simulink model "kinematics"  (Simulink 7.9)
settings: Solver=ode3  StartTime=0.0  StopTime=10.0  FixedStep=0.005  RelTol=1e-5
values from neighbouring files (symbols this model uses):
  initial_ee_eta = zeros(1,6)    [kinematic_parameters.m]
  initial_eta = [0,0,0,0,0,0]    [kinematic_parameters.m]
  initial_eta1 = initial_eta(1:3)    [kinematic_parameters.m]
  initial_eta2 = initial_eta(4:6)    [kinematic_parameters.m]
  initial_q = [0,20*d2r,-(20+25)*d2r,25*d2r,-90*d2r,0]    [kinematic_parameters.m]
  v_ee_c = [0.1,0,0,0,0.2,0]    [kinematic_parameters.m]
undefined symbols (not defined in the file or in its folder): a, alpha, d, qmax, qmin
libraries: simulink x3
settings Model: Creator=simena  LastModifiedBy=simena
settings OptimizationCC: EfficientMapNaN2IntZero=off
settings HardwareCC: TargetIntDivRoundTo=Zero  TargetEndianess=LittleEndian  TargetHWDeviceType=MATLAB Host  ProdEqTarget=off
settings CodeAppCC: MaxIdLength=128
settings GRTTargetCC: CombineOutputUpdateFcns=off  GRTInterface=on

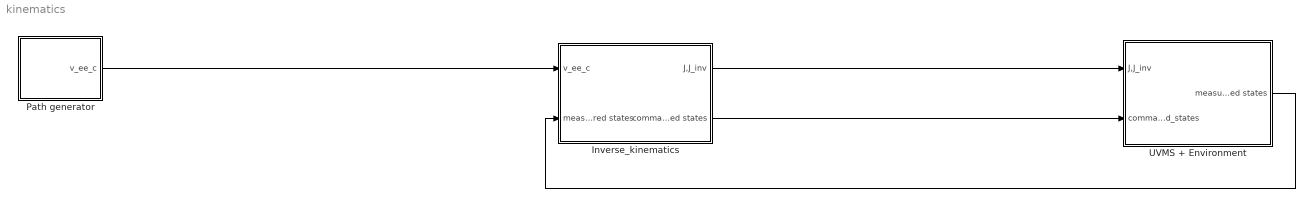
== system kinematics ==
  "Inverse_kinematics " : Subsystem
  Path generator : Subsystem
  UVMS + Environment : Subsystem
  wires:
  Path generator/1(v_ee_c) -> "Inverse_kinematics "/1(v_ee_c)
  "Inverse_kinematics "/1(J,J_inv) -> UVMS + Environment/1(J,J_inv)
  "Inverse_kinematics "/2(commanded states) -> UVMS + Environment/2(commanded_states)
  UVMS + Environment/1(measured states) -> "Inverse_kinematics "/2(measured states)

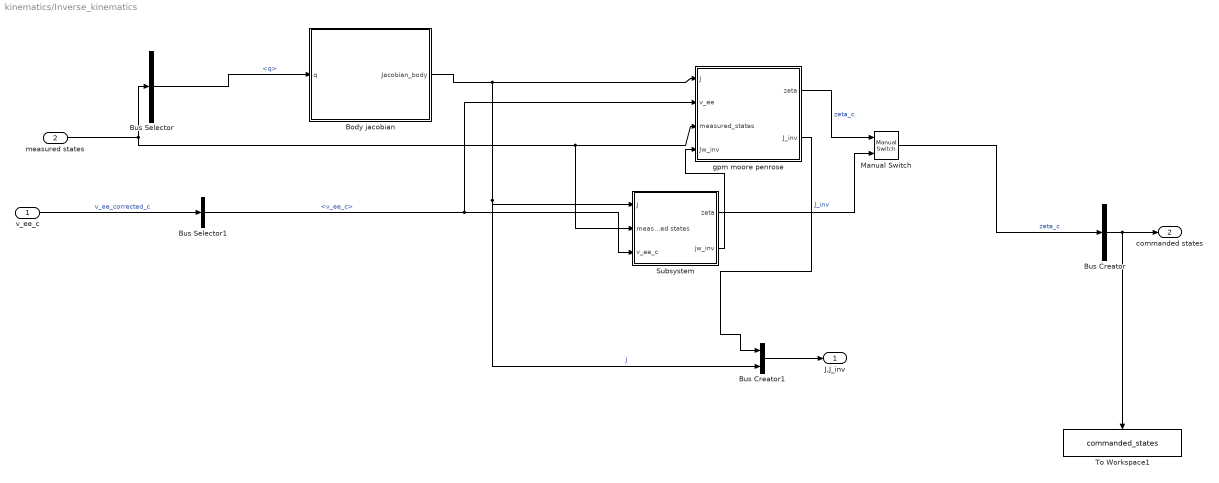
== system kinematics/Inverse_kinematics  ==
  v_ee_c : Inport
  measured states : Inport  Port=2
  Body jacobian : MATLAB Function  TreatAsAtomicUnit=on
  Bus Creator : BusCreator  Inputs=1
  Bus Creator1 : BusCreator  Inputs=2
  Bus Selector : BusSelector  OutputSignals=xi.q
  Bus Selector1 : BusSelector  OutputSignals=v_ee_c
  Manual Switch : simulink/Signal Routing/Manual Switch  sw=0  action=0  varsize=off
  Subsystem : Subsystem
  To Workspace1 : ToWorkspace  VariableName=commanded_states  SampleTime=-1  SaveFormat=Timeseries
  gpm moore penrose : Subsystem
  J,J_inv : Outport
  commanded states : Outport  Port=2
  wires:
  measured states/1 -> Bus Selector/1, gpm moore penrose/3(measured_states), Subsystem/2(measured states)
  Bus Creator/1 -> commanded states/1, To Workspace1/1
  Bus Creator1/1 -> J,J_inv/1
  gpm moore penrose/2(J_inv) -> Bus Creator1/1  "J_inv"
  v_ee_c/1 -> Bus Selector1/1  "v_ee_corrected_c"
  Body jacobian/1(Jacobian_body) -> gpm moore penrose/1(J), Bus Creator1/2, Subsystem/1(J)  "J"
  Bus Selector/1 -> Body jacobian/1(q)  "<q>"
  gpm moore penrose/1(zeta) -> Manual Switch/1  "zeta_c"
  Manual Switch/1 -> Bus Creator/1  "zeta_c"
  Subsystem/1(zeta) -> Manual Switch/2
  Bus Selector1/1 -> Subsystem/3(v_ee_c), gpm moore penrose/2(v_ee)  "<v_ee_c>"
  Subsystem/2(jw_inv) -> gpm moore penrose/4(Jw_inv)

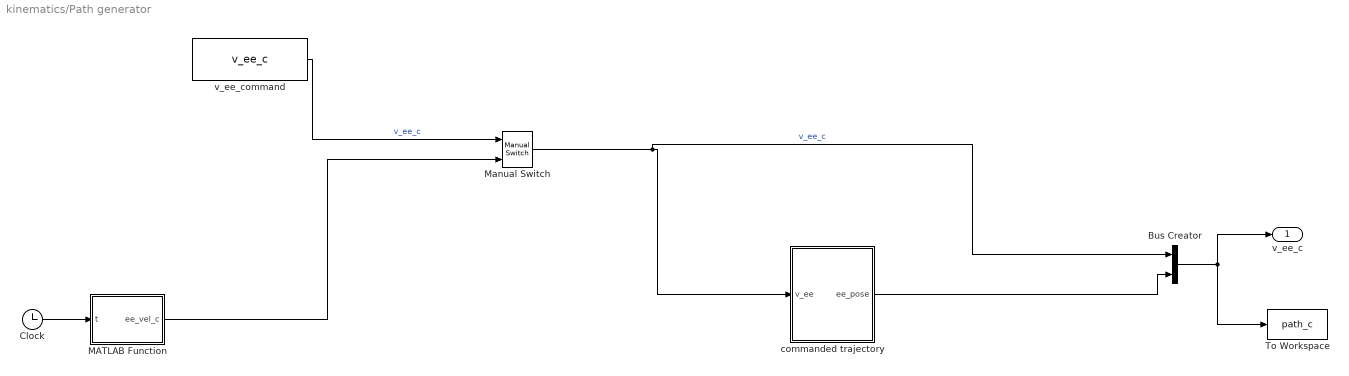
== system kinematics/Path generator ==
  Bus Creator : BusCreator  Inputs=2
  Clock : Clock
  MATLAB Function : MATLAB Function  TreatAsAtomicUnit=on
  Manual Switch : simulink/Signal Routing/Manual Switch  sw=0  action=0  varsize=off
  To Workspace : ToWorkspace  VariableName=path_c  SampleTime=-1  SaveFormat=Timeseries
  commanded trajectory : Subsystem
  v_ee_command : Constant  Value=v_ee_c
  v_ee_c : Outport
  wires:
  commanded trajectory/1(ee_pose) -> Bus Creator/2
  Bus Creator/1 -> v_ee_c/1, To Workspace/1
  v_ee_command/1 -> Manual Switch/1  "v_ee_c"
  Manual Switch/1 -> commanded trajectory/1(v_ee), Bus Creator/1  "v_ee_c"
  Clock/1 -> MATLAB Function/1(t)
  MATLAB Function/1(ee_vel_c) -> Manual Switch/2

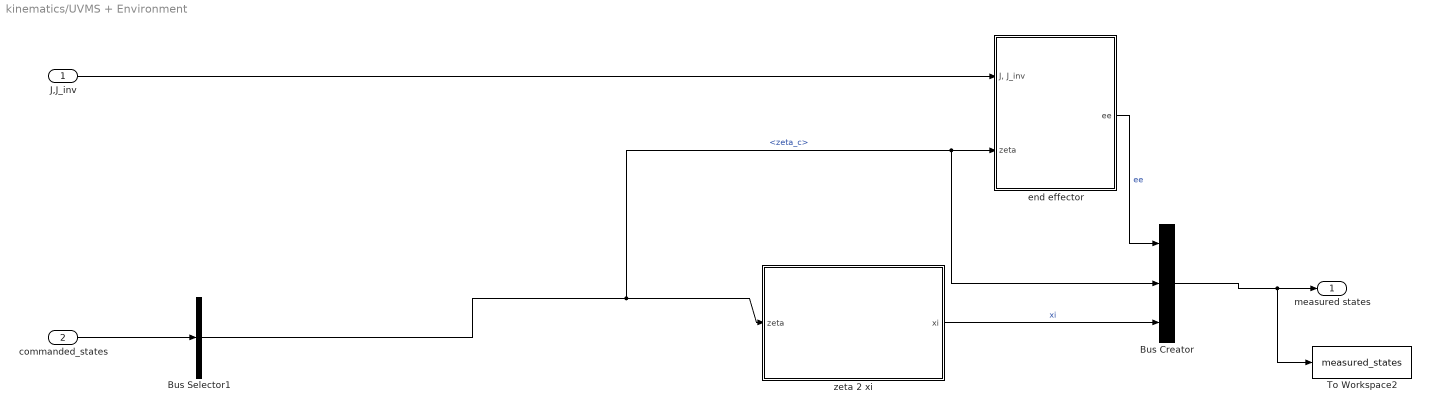
== system kinematics/UVMS + Environment ==
  J,J_inv : Inport
  commanded_states : Inport  Port=2
  Bus Creator : BusCreator  Inputs=3
  Bus Selector1 : BusSelector  OutputSignals=zeta_c
  To Workspace2 : ToWorkspace  VariableName=measured_states  SampleTime=-1  SaveFormat=Timeseries
  end effector : Subsystem
  zeta 2 xi : Subsystem
  measured states : Outport
  wires:
  zeta 2 xi/1(xi) -> Bus Creator/3  "xi"
  J,J_inv/1 -> end effector/1("J, J_inv")
  end effector/1(ee) -> Bus Creator/1  "ee"
  commanded_states/1 -> Bus Selector1/1
  Bus Creator/1 -> measured states/1, To Workspace2/1
  Bus Selector1/1 -> zeta 2 xi/1(zeta), end effector/2(zeta), Bus Creator/2  "<zeta_c>"

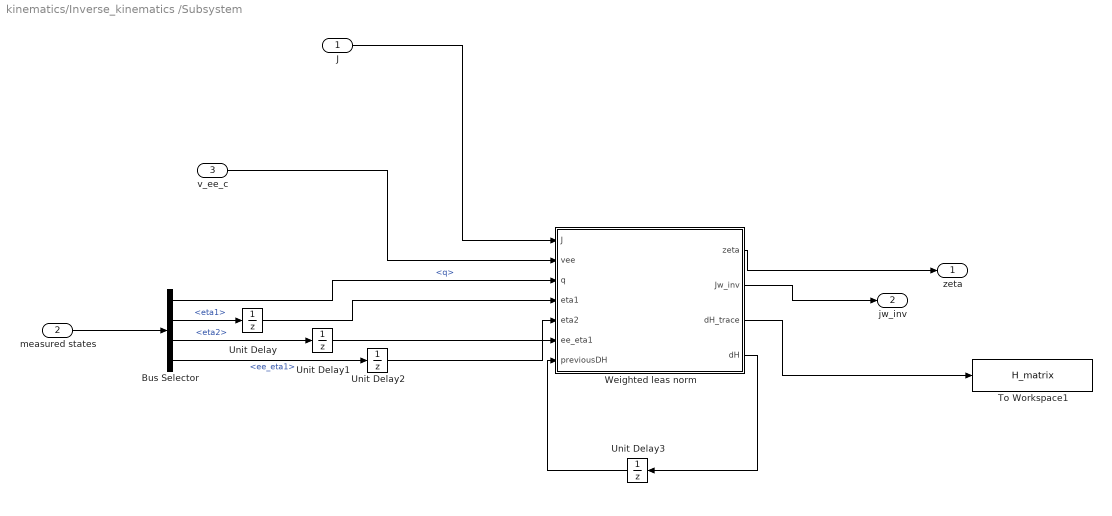
== system kinematics/Inverse_kinematics /Subsystem ==
  J : Inport
  measured states : Inport  Port=2
  v_ee_c : Inport  Port=3
  Bus Selector : BusSelector  OutputSignals=xi.q,xi.eta1,xi.eta2,ee.ee_eta1
  To Workspace1 : ToWorkspace  VariableName=H_matrix  SampleTime=-1  SaveFormat=Timeseries
  Unit Delay : UnitDelay  X0=initial_eta1  SampleTime=-1
  Unit Delay1 : UnitDelay  X0=initial_eta2  SampleTime=-1
  Unit Delay2 : UnitDelay  X0=initial_ee_eta(4:6)  SampleTime=-1
  Unit Delay3 : UnitDelay  X0=zeros(12,12)  SampleTime=-1
  Weighted leas norm : MATLAB Function  TreatAsAtomicUnit=on
  zeta : Outport
  jw_inv : Outport  Port=2
  wires:
  Weighted leas norm/1(zeta) -> zeta/1
  J/1 -> Weighted leas norm/1(J)
  measured states/1 -> Bus Selector/1
  v_ee_c/1 -> Weighted leas norm/2(vee)
  Bus Selector/1 -> Weighted leas norm/3(q)  "<q>"
  Bus Selector/2 -> Unit Delay/1  "<eta1>"
  Bus Selector/3 -> Unit Delay1/1  "<eta2>"
  Bus Selector/4 -> Unit Delay2/1  "<ee_eta1>"
  Unit Delay/1 -> Weighted leas norm/4(eta1)
  Unit Delay1/1 -> Weighted leas norm/5(eta2)
  Unit Delay2/1 -> Weighted leas norm/6(ee_eta1)
  Weighted leas norm/2(Jw_inv) -> jw_inv/1
  Weighted leas norm/3(dH_trace) -> To Workspace1/1
  Weighted leas norm/4(dH) -> Unit Delay3/1
  Unit Delay3/1 -> Weighted leas norm/7(previousDH)

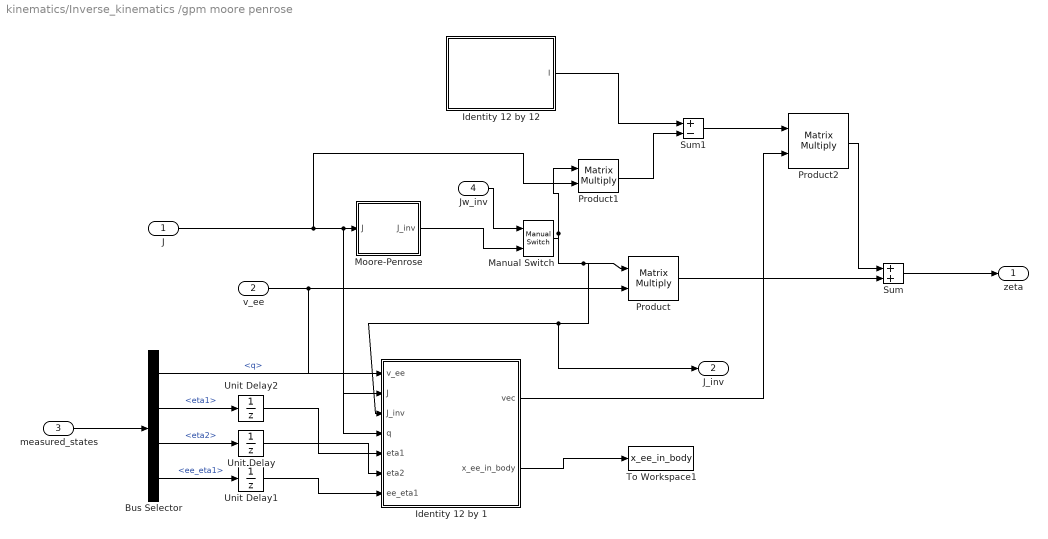
== system kinematics/Inverse_kinematics /gpm moore penrose ==
  J : Inport
  v_ee : Inport  Port=2
  measured_states : Inport  Port=3
  Jw_inv : Inport  Port=4
  Bus Selector : BusSelector  OutputSignals=xi.q,xi.eta1,xi.eta2,ee.ee_eta1
  Identity 12 by 1 : MATLAB Function  TreatAsAtomicUnit=on
  Identity 12 by 12 : MATLAB Function  TreatAsAtomicUnit=on
  Manual Switch : simulink/Signal Routing/Manual Switch  sw=1  action=0  varsize=off
  Moore-Penrose : MATLAB Function  TreatAsAtomicUnit=on
  Product : Product  Multiplication=Matrix(*)  RndMeth=Zero
  Product1 : Product  Multiplication=Matrix(*)  RndMeth=Zero
  Product2 : Product  Multiplication=Matrix(*)  RndMeth=Zero
  Sum : Sum
  Sum1 : Sum  Inputs=+-
  To Workspace1 : ToWorkspace  VariableName=x_ee_in_body  SampleTime=-1  SaveFormat=Timeseries
  Unit Delay : UnitDelay  X0=initial_eta2  SampleTime=-1
  Unit Delay1 : UnitDelay  X0=initial_ee_eta(1:3)  SampleTime=-1
  Unit Delay2 : UnitDelay  X0=initial_eta1  SampleTime=-1
  zeta : Outport
  J_inv : Outport  Port=2
  wires:
  Product/1 -> Sum/2
  Identity 12 by 12/1(I) -> Sum1/1
  Product1/1 -> Sum1/2
  Sum1/1 -> Product2/1
  Product2/1 -> Sum/1
  v_ee/1 -> Product/2, Identity 12 by 1/1(v_ee)
  Sum/1 -> zeta/1
  Identity 12 by 1/1(vec) -> Product2/2
  measured_states/1 -> Bus Selector/1
  Bus Selector/2 -> Unit Delay2/1  "<eta1>"
  Bus Selector/4 -> Unit Delay1/1  "<ee_eta1>"
  Bus Selector/3 -> Unit Delay/1  "<eta2>"
  Bus Selector/1 -> Identity 12 by 1/4(q)  "<q>"
  Unit Delay2/1 -> Identity 12 by 1/5(eta1)
  Unit Delay/1 -> Identity 12 by 1/6(eta2)
  Unit Delay1/1 -> Identity 12 by 1/7(ee_eta1)
  Jw_inv/1 -> Manual Switch/1
  Moore-Penrose/1(J_inv) -> Manual Switch/2
  Manual Switch/1 -> Product1/1, Product/1, Identity 12 by 1/3(J_inv), J_inv/1
  J/1 -> Moore-Penrose/1(J), Identity 12 by 1/2(J), Product1/2
  Identity 12 by 1/2(x_ee_in_body) -> To Workspace1/1

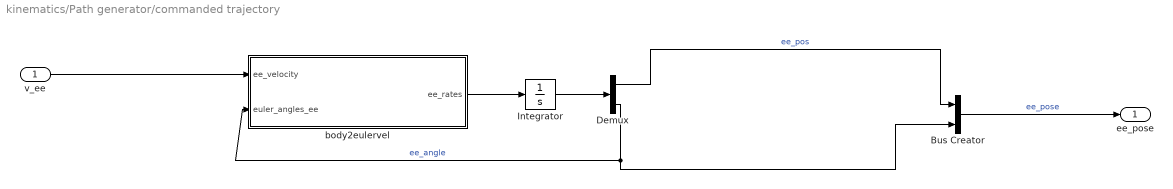
== system kinematics/Path generator/commanded trajectory ==
  v_ee : Inport
  Bus Creator : BusCreator  Inputs=2
  Demux : Demux  Outputs=2
  Integrator : Integrator  InitialCondition=initial_ee_eta
  body2eulervel : MATLAB Function  TreatAsAtomicUnit=on
  ee_pose : Outport
  wires:
  v_ee/1 -> body2eulervel/1(ee_velocity)
  body2eulervel/1(ee_rates) -> Integrator/1
  Integrator/1 -> Demux/1
  Demux/1 -> Bus Creator/1  "ee_pos"
  Demux/2 -> body2eulervel/2(euler_angles_ee), Bus Creator/2  "ee_angle"
  Bus Creator/1 -> ee_pose/1  "ee_pose"

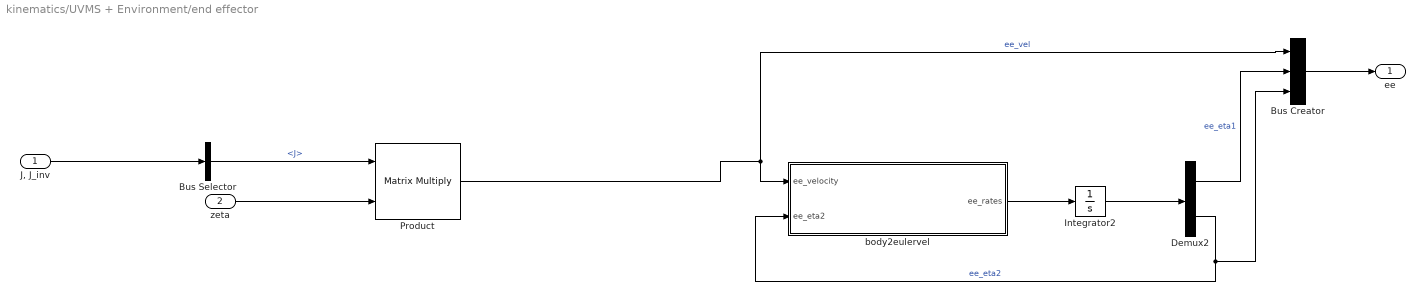
== system kinematics/UVMS + Environment/end effector ==
  "J, J_inv" : Inport
  zeta : Inport  Port=2
  Bus Creator : BusCreator  Inputs=3
  Bus Selector : BusSelector  OutputSignals=J
  Demux2 : Demux  Outputs=2
  Integrator2 : Integrator  InitialCondition=initial_ee_eta
  Product : Product  Multiplication=Matrix(*)  RndMeth=Zero
  body2eulervel : MATLAB Function  TreatAsAtomicUnit=on
  ee : Outport
  wires:
  zeta/1 -> Product/2
  Demux2/2 -> body2eulervel/2(ee_eta2), Bus Creator/3  "ee_eta2"
  Integrator2/1 -> Demux2/1
  body2eulervel/1(ee_rates) -> Integrator2/1
  Product/1 -> body2eulervel/1(ee_velocity), Bus Creator/1  "ee_vel"
  Demux2/1 -> Bus Creator/2  "ee_eta1"
  Bus Creator/1 -> ee/1
  "J, J_inv"/1 -> Bus Selector/1
  Bus Selector/1 -> Product/1  "<J>"

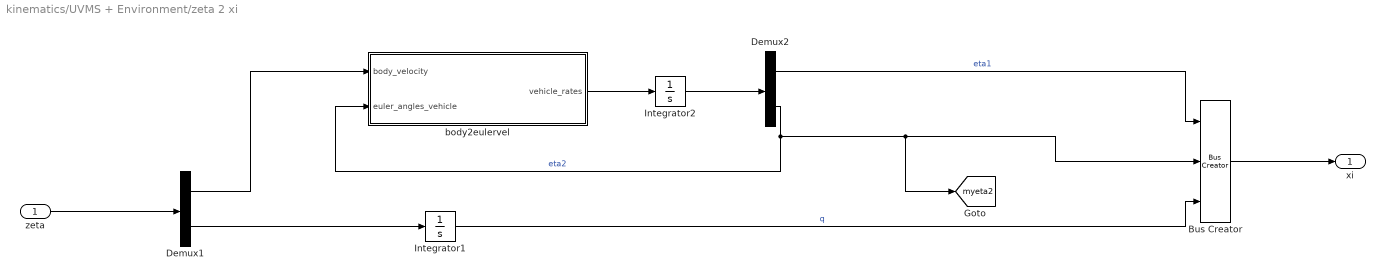
== system kinematics/UVMS + Environment/zeta 2 xi ==
  zeta : Inport
  Bus Creator : BusCreator  Inputs=3
  Demux1 : Demux  Outputs=2
  Demux2 : Demux  Outputs=2
  Integrator1 : Integrator  InitialCondition=initial_q
  Integrator2 : Integrator  InitialCondition=initial_eta
  body2eulervel : MATLAB Function  TreatAsAtomicUnit=on
  xi : Outport
  tag scope: myeta2=global
  wires:
  Demux2/1 -> Bus Creator/1  "eta1"
  Demux2/2 -> body2eulervel/2(euler_angles_vehicle), Bus Creator/2, [myeta2]  "eta2"
  Integrator2/1 -> Demux2/1
  body2eulervel/1(vehicle_rates) -> Integrator2/1
  Integrator1/1 -> Bus Creator/3  "q"
  Demux1/1 -> body2eulervel/1(body_velocity)
  Demux1/2 -> Integrator1/1
  zeta/1 -> Demux1/1
  Bus Creator/1 -> xi/1

== matlab function Inverse_kinematics /gpm moore penrose/Identity 12 by 12 ==
  data: I output double
function I = Identity_mat()
    %#codegen
    I=eye(12);
end

== matlab function Inverse_kinematics /Body jacobian ==
  data: q input double; Jacobian_body output double
function Jacobian_body = fcn(q)
    %#codegen
    
    Jacobian_body=zeros(6,12);
    coder.extrinsic('body_jacobian');
    newq=zeros(1,6);
    newq=q;
    Jacobian_body=body_jacobian(newq);
end

== matlab function Path generator/MATLAB Function ==
  data: t input double; ee_vel_c output double
function ee_vel_c = fcn(t)
%#codegen
ee_vel_c = zeros(6,1);
xvel=0.8*cos(t);
zvel=0.2*sin(t);
ee_vel_c(1)=xvel;
ee_vel_c(3)=zvel;
end

== matlab function Inverse_kinematics /gpm moore penrose/Moore-Penrose ==
  data: J input double; J_inv output double
function J_inv = moore_penrose(J)
    %#codegen
       
    J_inv=zeros(12,6);
    J_inv = pinv(J);      
end

== matlab function UVMS + Environment/end effector/body2eulervel ==
  data: ee_velocity input double; ee_rates output double; ee_eta2 input double
function ee_rates = fcn(ee_velocity, ee_eta2)                       
    %#codegen
    coder.extrinsic('analytical_jacobian');
    J=analytical_jacobian(ee_eta2);

    ee_rates = zeros(6,1);
    ee_rates=J*ee_velocity;
end

== matlab function Inverse_kinematics /Subsystem/Weighted leas norm ==
  data: J input double; zeta output double; vee input double; q input double; eta1 input double; eta2 input double; ee_eta1 input double; qmin parameter double size=6; qmax parameter double size=6; d parameter double size=6; a parameter double size=6; alpha parameter double size=6; Jw_inv output double; dH_trace output double; dH output double; previousDH input double
function [zeta, Jw_inv,dH_trace,dH] = wln(J,vee,q, eta1,eta2,ee_eta1,qmin, qmax,d,a,alpha,previousDH)
%#codegen
    
    dH_trace=zeros(12,1);
    dH_prev=previousDH;
    % generate weighting matrix
    dH=eye(12);
    eta2_w_factors=[4000,4000,10];
    
    
    % roll
    roll_max=80*(pi/180);
    roll_min=-80*(pi/180);
    temp= 1 + abs((((roll_max-roll_min).^2)*(2*eta2(1)-roll_max-roll_min)) / ((4*(roll_max-eta2(1)).^2) * ((eta2(1)-roll_min).^2))) + (300*eta2(1)).^4;
    
    dH(4,4)=10+temp;
   
    
    % pitch
    pitch_max=80*(pi/180);
    pitch_min=-80*(pi/180);
    temp= 1 + abs((((pitch_max-pitch_min).^2)*(2*eta2(2)-pitch_max-pitch_min)) / ((4*(pitch_max-eta2(2)).^2) * ((eta2(2)-pitch_min).^2)))  + (50*eta2(2)).^2;
    
    dH(5,5)=10+temp;
    
%     % x direction
    coder.extrinsic('ee_in_vechicle_frame');
    
    ee_pos=ee_in_vehicle_frame(q,d,a,alpha);
    
    xmax=1.9;
    xmin=0.4;
    x=ee_pos(1);
    dev_x = abs(x-2.2);
    stddev_x=0.2;
    temp=200 + 2000*exp(- (dev_x.^2)./(2*stddev_x.^2));
    %temp= 1 + abs((((xmax-xmin).^2)*(2*x-xmax-xmin)) / ((4*(xmax-x).^2) * ((x-xmin).^2)))  + (400*x).^4;
    dH(1,1)=760;
    
    for i=4:6
        dH(i,i)=470;
    end

    
   
    
       
    
    %vehicle position rates
    for i=2:3
        dH(i,i)=400;
    end
    
    
    % link joints
    for i=1:6
        temp = abs((((qmax(i)-qmin(i)).^2)*(2*q(i)-qmax(i)-qmin(i))) / ((4*(qmax(i)-q(i)).^2) * ((q(i)-qmin(i)).^2)));
        if (temp-previousDH(i+6,i+6))<0 
            dH(i+6,i+6)=0;
        else
            dH(i+6,i+6)=temp;
        end
                
    end
    
    % return dH
    
    
    
    
    
    
    
    
    
    
    %% generate the matrixes
    W=eye(12);
    W=W+dH;
    
    Wi=inv(W);
    Jt=J';
    inv_prod = inv(J*Wi*Jt);
    J_inv=zeros(12,6);
    J_inv=Wi*Jt*inv_prod;  
    Jw_inv=J_inv;   
    zeta = J_inv(1:12,1:6)*vee;
    
    
    for i=1:12
        dH_trace(i)=dH(i,i);
    end
    
end









    
    
    
    




















function dH = generateDHMatrix(q,eta1,eta2,ee_eta1,qmin,qmax)
        
    
    
    
end

== matlab function Path generator/commanded trajectory/body2eulervel ==
  data: ee_velocity input double; ee_rates output double; euler_angles_ee input double
function ee_rates = fcn(ee_velocity, euler_angles_ee)                       
    %#codegen
    coder.extrinsic('analytical_jacobian');
    J=analytical_jacobian(euler_angles_ee);

    ee_rates = zeros(6,1);
    ee_rates=J*ee_velocity;
end

== matlab function Inverse_kinematics /gpm moore penrose/Identity 12 by 1 ==
  data: v_ee input double; J input double; J_inv input double; vec output double; q input double; eta1 input double; eta2 input double; ee_eta1 input double; qmin parameter double size=6; qmax parameter double size=6; d parameter double size=6; a parameter double size=6; alpha parameter double size=6; x_ee_in_body output double
function [vec,x_ee_in_body] = H_grad(v_ee,J,J_inv,q,eta1,eta2,ee_eta1,qmin,qmax,d,a,alpha)
    %#codegen
%     qmin=qlimits.qmin;
%     qmax=qlimits.qmax;
    coder.extrinsic('ee_in_vechicle_frame');
    ee_pos=ee_in_vehicle_frame(q,d,a,alpha);
    
    

    h_q = zeros(6,1);
    h_phi = (2*eta2(1))*100;
    h_theta =(2*eta2(2))*50;
    h_x = -(5*(1*ee_pos(1)-1.3));
    h_z = -(20*ee_pos(3));
    
    for i=1:6
        h_q(i)= (1/4)*(-(qmax(i) - qmin(i)).^2)/((-q(i) + qmax(i))*(q(i) - qmin(i)).^2) + (qmax(i) - qmin(i)).^2/((-q(i) + qmax(i)).^2*(q(i) - qmin(i)));       
    end
    I=eye(12);
    
    
    
    % x-direction 
    coder.extrinsic('ee_in_vechicle_frame');
    
    ee_pos=ee_in_vehicle_frame(q,d,a,alpha);
    x=ee_pos(1);
    
    if x > 2.1
        x_b_vel=2*(x-2.1).^2;
    elseif x < 1.5
        x_b_vel=-2*(x-1.5).^2;
    else
        x_b_vel=0;   
    end
    
    %temp= 1 + abs((((xmax-xmin).^2)*(2*x-xmax-xmin)) / ((4*(xmax-x).^2) * ((x-xmin).^2)))  + (400*x).^4;
    
    x_ee_in_body=x;
    
    
    
    vec=zeros(12,1);
    %vec(7:12)=h_q;
%     vec(4)=h_phi;
     vec(1)=x_b_vel;
%     vec(5)=h_theta;
%     %k=-((2-norm(J_inv*v_ee)))/(norm(I-J_inv*J)*norm((I-J_inv*J)*vec));
     k=0.4;
     vec=k*vec;
%     %vec(1)=0.4;
    
end

== matlab function UVMS + Environment/zeta 2 xi/body2eulervel ==
  data: body_velocity input double; vehicle_rates output double; euler_angles_vehicle input double
function vehicle_rates = fcn(body_velocity, euler_angles_vehicle)                       
    %#codegen
    coder.extrinsic('analytical_jacobian');
    J=analytical_jacobian(euler_angles_vehicle);

    vehicle_rates = zeros(6,1);
    vehicle_rates=J*body_velocity;
end
